simulink model "NonlinearBlockLibraryObserver"  (R2019b)
settings: Solver=VariableStepAuto  StartTime=0.0  StopTime=30.0  RelTol=1e-3
libraries: eeLuenbergerObserver x2
settings Model: Creator=marko  LastModifiedBy=marko

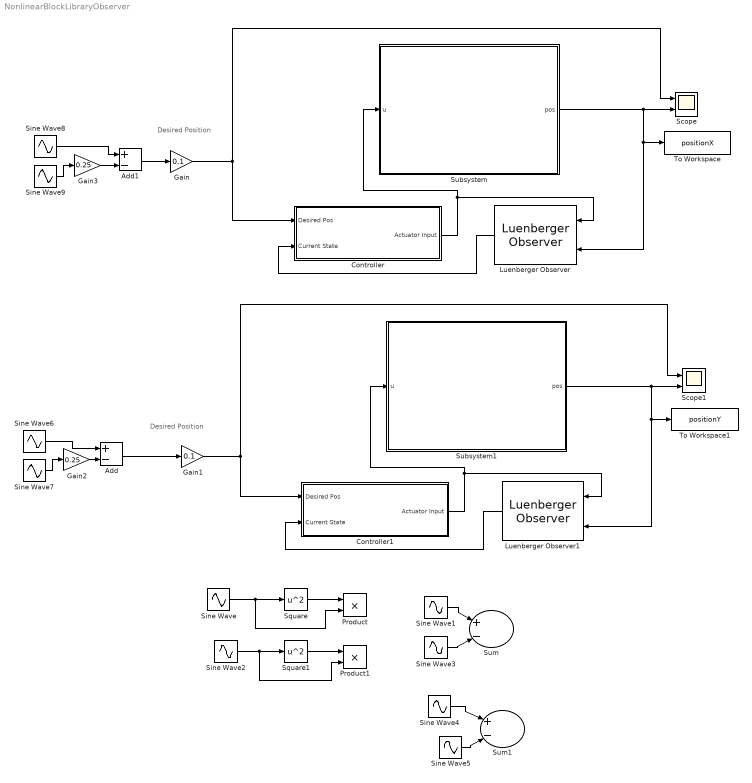
== system NonlinearBlockLibraryObserver ==
  note: Desired Position
  note: Desired Position
  Add : Sum  Inputs=+-
  Add1 : Sum  Inputs=+-
  Controller : Subsystem
  Controller1 : Subsystem
  Gain : Gain  Gain=0.1
  Gain1 : Gain  Gain=0.1
  Gain2 : Gain  Gain=0.25
  Gain3 : Gain  Gain=0.25
  Luenberger Observer : eeLuenbergerObserver/Luenberger Observer  StateSpaceType=Continuous-time  Ad=1  Bd=1  Cd=1  Dd=1  A=[0 1 0 0; 0 -1 -9.8 0; 0 0 0 1; -0.98/(0.33) 0 0 -0.1/(0.33)]  B=[0; 0; 0; 3]  C=[1 0 0 0]  D=0  ObserverDesign=Desired eigenvalues  Ld=1  DesiredEigenvalues=[-40, -50, -60, -70]  x0=[0; 0; 0; 0]  Tsd=0.01  Ts=0.01
      settings: SourceProductName=Simscape Electrical  SourceProductBaseCode=PS
  Luenberger Observer1 : eeLuenbergerObserver/Luenberger Observer  StateSpaceType=Continuous-time  Ad=1  Bd=1  Cd=1  Dd=1  A=[0 1 0 0; 0 -1 -9.8 0; 0 0 0 1; -0.98/(0.33) 0 0 -0.1/(0.33)]  B=[0; 0; 0; 3]  C=[1 0 0 0]  D=0  ObserverDesign=Desired eigenvalues  Ld=1  DesiredEigenvalues=[-40, -50, -60, -70]  x0=[0; 0; 0; 0]  Tsd=0.01  Ts=0.01
      settings: SourceProductName=Simscape Electrical  SourceProductBaseCode=PS
  Product : Product
  Product1 : Product
  Scope : Scope  NumInputPorts=2
  Scope1 : Scope  NumInputPorts=2
  Sine Wave : Sin  SampleTime=0
  Sine Wave1 : Sin  Amplitude=2  SampleTime=0
  Sine Wave2 : Sin  Phase=pi/2  SampleTime=0
  Sine Wave3 : Sin  Frequency=2  SampleTime=0
  Sine Wave4 : Sin  Amplitude=2  Phase=pi/2  SampleTime=0
  Sine Wave5 : Sin  Frequency=2  Phase=pi/2  SampleTime=0
  Sine Wave6 : Sin  Amplitude=1.25  SampleTime=0
  Sine Wave7 : Sin  Frequency=5  SampleTime=0
  Sine Wave8 : Sin  Amplitude=1.25  Phase=pi/2  SampleTime=0
  Sine Wave9 : Sin  Frequency=5  Phase=pi/2  SampleTime=0
  Square : Math  Operator=square  SignedPower=off  SaturateOnIntegerOverflow=on
  Square1 : Math  Operator=square  SignedPower=off  SaturateOnIntegerOverflow=on
  Subsystem : Subsystem
  Subsystem1 : Subsystem
  Sum : Sum  Inputs=|+-|
  Sum1 : Sum  Inputs=|+-|
  To Workspace : ToWorkspace  VariableName=positionX  SampleTime=-1
  To Workspace1 : ToWorkspace  VariableName=positionY  SampleTime=-1
  wires:
  Subsystem/1(pos) -> Scope/2, To Workspace/1, Luenberger Observer/2
  Controller/1(Actuator Input) -> Subsystem/1(u), Luenberger Observer/1
  Luenberger Observer/1 -> Controller/2(Current State)
  Controller1/1(Actuator Input) -> Subsystem1/1(u), Luenberger Observer1/1
  Luenberger Observer1/1 -> Controller1/2(Current State)
  Subsystem1/1(pos) -> Scope1/2, To Workspace1/1, Luenberger Observer1/2
  Sine Wave/1 -> Product/2, Square/1
  Square/1 -> Product/1
  Sine Wave2/1 -> Product1/2, Square1/1
  Square1/1 -> Product1/1
  Gain/1 -> Controller/1(Desired Pos), Scope/1
  Gain1/1 -> Controller1/1(Desired Pos), Scope1/1
  Add/1 -> Gain1/1
  Add1/1 -> Gain/1
  Sine Wave1/1 -> Sum/1
  Sine Wave3/1 -> Sum/2
  Sine Wave5/1 -> Sum1/2
  Sine Wave4/1 -> Sum1/1
  Sine Wave6/1 -> Add/1
  Gain2/1 -> Add/2
  Sine Wave7/1 -> Gain2/1
  Sine Wave9/1 -> Gain3/1
  Sine Wave8/1 -> Add1/1
  Gain3/1 -> Add1/2

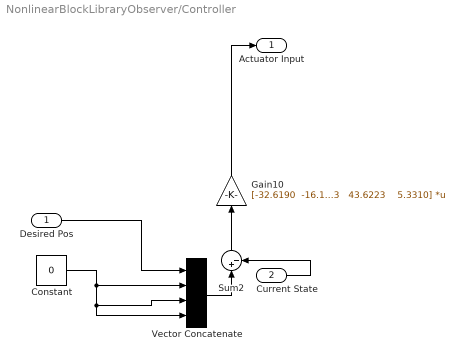
== system NonlinearBlockLibraryObserver/Controller ==
  Desired Pos : Inport
  Current State : Inport  Port=2
  Constant : Constant  Value=0
  Gain10 : Gain  Gain="[-32.6190  -16.1083   43.6223    5.3310]"  Multiplication=Matrix(K*u)
  Sum2 : Sum  Inputs=|+-
  Vector Concatenate : Concatenate  NumInputs=4
  Actuator Input : Outport
  wires:
  Desired Pos/1 -> Vector Concatenate/1
  Gain10/1 -> Actuator Input/1
  Constant/1 -> Vector Concatenate/2, Vector Concatenate/4, Vector Concatenate/3
  Current State/1 -> Sum2/2
  Sum2/1 -> Gain10/1
  Vector Concatenate/1 -> Sum2/1

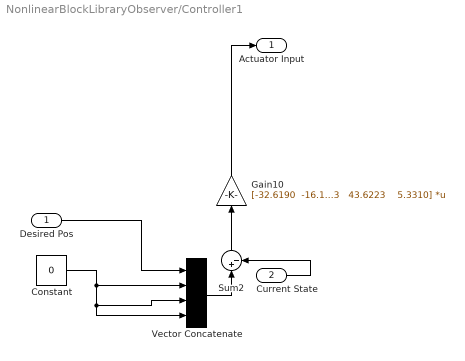
== system NonlinearBlockLibraryObserver/Controller1 ==
  Desired Pos : Inport
  Current State : Inport  Port=2
  Constant : Constant  Value=0
  Gain10 : Gain  Gain="[-32.6190  -16.1083   43.6223    5.3310]"  Multiplication=Matrix(K*u)
  Sum2 : Sum  Inputs=|+-
  Vector Concatenate : Concatenate  NumInputs=4
  Actuator Input : Outport
  wires:
  Desired Pos/1 -> Vector Concatenate/1
  Gain10/1 -> Actuator Input/1
  Constant/1 -> Vector Concatenate/2, Vector Concatenate/4, Vector Concatenate/3
  Current State/1 -> Sum2/2
  Sum2/1 -> Gain10/1
  Vector Concatenate/1 -> Sum2/1

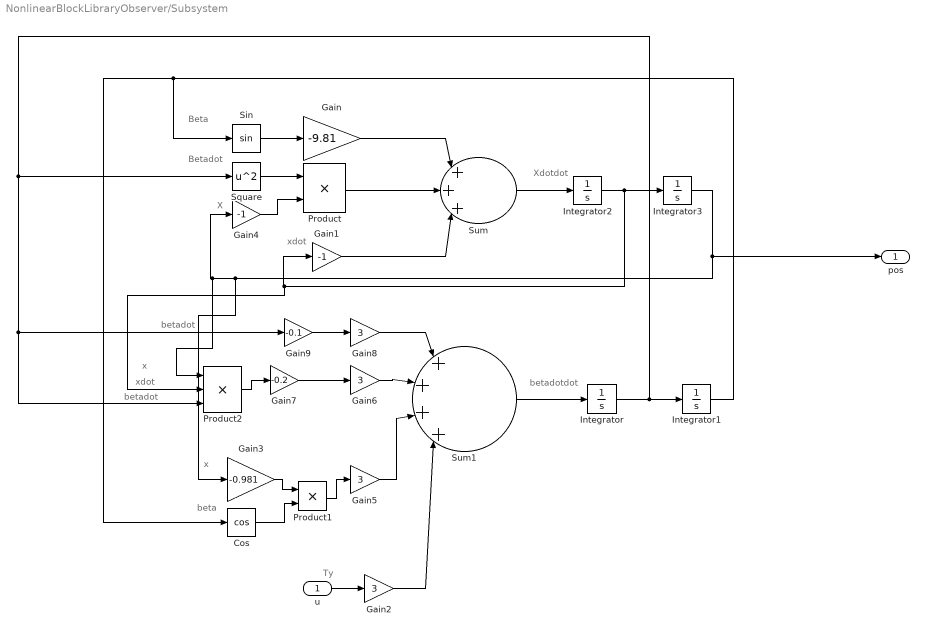
== system NonlinearBlockLibraryObserver/Subsystem ==
  note: betadotdot
  note: betadot
  note: betadot
  note: xdot
  note: x
  note: beta
  note: x
  note: Ty
  note: xdot
  note: X
  note: Betadot
  note: Beta
  note: Xdotdot
  u : Inport
  Cos : Trigonometry  Operator=cos
  Gain : Gain  Gain=-9.81
  Gain1 : Gain  Gain=-1
  Gain{2,5..6,8} (4 alike) : Gain  Gain=3
  Gain3 : Gain  Gain=-0.981
  Gain4 : Gain  Gain=-1
  Gain7 : Gain  Gain=-0.2
  Gain9 : Gain  Gain=-0.1
  Integrator{,1..3} (4 alike) : Integrator
  Product : Product
  Product1 : Product
  Product2 : Product  Inputs=3
  Sin : Trigonometry
  Square : Math  Operator=square  SignedPower=off  SaturateOnIntegerOverflow=on
  Sum : Sum  Inputs=|+++|
  Sum1 : Sum  Inputs=|++++|
  pos : Outport
  wires:
  Gain2/1 -> Sum1/4
  Gain8/1 -> Sum1/1
  Sum1/1 -> Integrator/1
  Integrator3/1 -> pos/1, Gain3/1, Product2/1, Gain4/1
  Product1/1 -> Gain5/1
  Gain1/1 -> Sum/3
  Product/1 -> Sum/2
  Gain4/1 -> Product/2
  Sum/1 -> Integrator2/1
  Square/1 -> Product/1
  Gain3/1 -> Product1/1
  Gain6/1 -> Sum1/2
  Gain9/1 -> Gain8/1
  Gain/1 -> Sum/1
  Cos/1 -> Product1/2
  Integrator/1 -> Gain9/1, Product2/3, Square/1, Integrator1/1
  Integrator1/1 -> Cos/1, Sin/1
  Gain5/1 -> Sum1/3
  Gain7/1 -> Gain6/1
  Sin/1 -> Gain/1
  Integrator2/1 -> Product2/2, Gain1/1, Integrator3/1
  Product2/1 -> Gain7/1
  u/1 -> Gain2/1

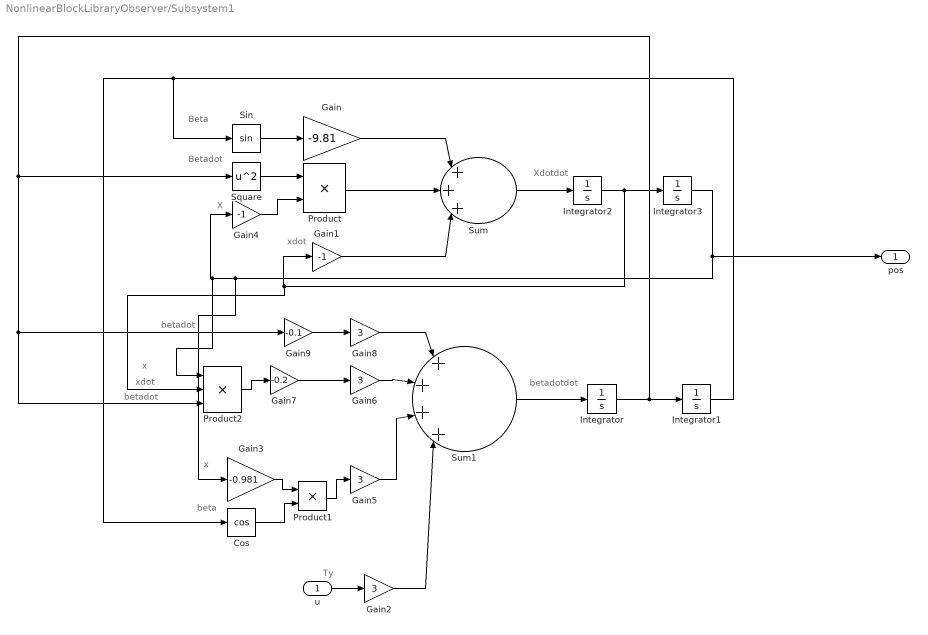
== system NonlinearBlockLibraryObserver/Subsystem1 ==
  note: betadotdot
  note: betadot
  note: betadot
  note: xdot
  note: x
  note: beta
  note: x
  note: Ty
  note: xdot
  note: X
  note: Betadot
  note: Beta
  note: Xdotdot
  u : Inport
  Cos : Trigonometry  Operator=cos
  Gain : Gain  Gain=-9.81
  Gain1 : Gain  Gain=-1
  Gain{2,5..6,8} (4 alike) : Gain  Gain=3
  Gain3 : Gain  Gain=-0.981
  Gain4 : Gain  Gain=-1
  Gain7 : Gain  Gain=-0.2
  Gain9 : Gain  Gain=-0.1
  Integrator{,1..3} (4 alike) : Integrator
  Product : Product
  Product1 : Product
  Product2 : Product  Inputs=3
  Sin : Trigonometry
  Square : Math  Operator=square  SignedPower=off  SaturateOnIntegerOverflow=on
  Sum : Sum  Inputs=|+++|
  Sum1 : Sum  Inputs=|++++|
  pos : Outport
  wires:
  Gain2/1 -> Sum1/4
  Gain8/1 -> Sum1/1
  Sum1/1 -> Integrator/1
  Integrator3/1 -> pos/1, Gain3/1, Product2/1, Gain4/1
  Product1/1 -> Gain5/1
  Gain1/1 -> Sum/3
  Product/1 -> Sum/2
  Gain4/1 -> Product/2
  Sum/1 -> Integrator2/1
  Square/1 -> Product/1
  Gain3/1 -> Product1/1
  Gain6/1 -> Sum1/2
  Gain9/1 -> Gain8/1
  Gain/1 -> Sum/1
  Cos/1 -> Product1/2
  Integrator/1 -> Gain9/1, Product2/3, Square/1, Integrator1/1
  Integrator1/1 -> Cos/1, Sin/1
  Gain5/1 -> Sum1/3
  Gain7/1 -> Gain6/1
  Sin/1 -> Gain/1
  Integrator2/1 -> Product2/2, Gain1/1, Integrator3/1
  Product2/1 -> Gain7/1
  u/1 -> Gain2/1
